simulink library "ros2lib"  (R2022a)
settings: Solver=ode45  StartTime=0.0  StopTime=10.0  RelTol=1e-3  EnableMultiTasking=on
undefined symbols (not defined in the file or in its folder): coder, count, data, data_SL_Info, datatype, encoding, encoding_SL_Info, fields, fields_SL_Info, height, name, name_SL_Info, offset, point_step, ros, row_step, width
settings Model: Creator=The MathWorks, Inc.  LastModifiedBy=The MathWorks, Inc.
settings SolverCC: AlgebraicLoopSolver=TrustRegion  MaxZcPerStep=1
settings DataIOCC: LimitDataPoints=on  SaveFormat=Array  ReturnWorkspaceOutputs=off
settings OptimizationCC: LifeSpan=inf
settings DebuggingCC: SolverPrmCheckMsg=warning  UnconnectedInputMsg=warning  UnconnectedOutputMsg=warning  UnconnectedLineMsg=warning  AllowSymbolicDim=off  PregeneratedLibrarySubsystemCodeDiagnostic=none  SFUnexpectedBacktrackingDiag=warning  SFNoUnconditionalDefaultTransitionDiag=warning  SFExecutionAtInitializationDiag=none  SFMachineParentedDataDiag=warning  ArithmeticOperatorsInVariantConditions=warning
settings HardwareCC: ProdBitPerPointer=32  ProdBitPerSizeT=32  ProdBitPerPtrDiffT=32  ProdLargestAtomicFloat=None  ProdIntDivRoundTo=Undefined  ProdEndianess=Unspecified  ProdWordSize=32  ProdHWDeviceType=32-bit Generic
settings ModelReferenceCC: PropagateSignalLabelsOutOfModel=off
settings SFSimCC: SimUseLocalCustomCode=off
settings RTWCC: RTWUseLocalCustomCode=off  DLArmComputeVersion=19.05
settings CodeAppCC: StateflowObjectComments=on
settings GRTTargetCC: TargetLangStandard=C89/C90 (ANSI)
settings ConfigComp: CovScope=ReferencedModels  CovMetricSettings=dw  CovSaveCumulativeToWorkspaceVar=on  CovSaveSingleToWorkspaceVar=on  CovExternalEMLEnable=off  CovSFcnEnable=off

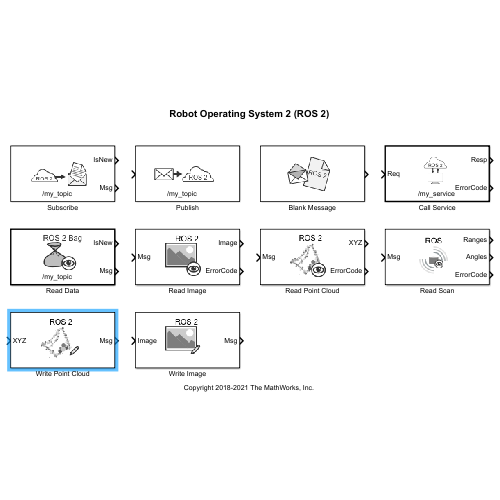
[thumbnail: Simulink's stored preview of the top-level diagram]
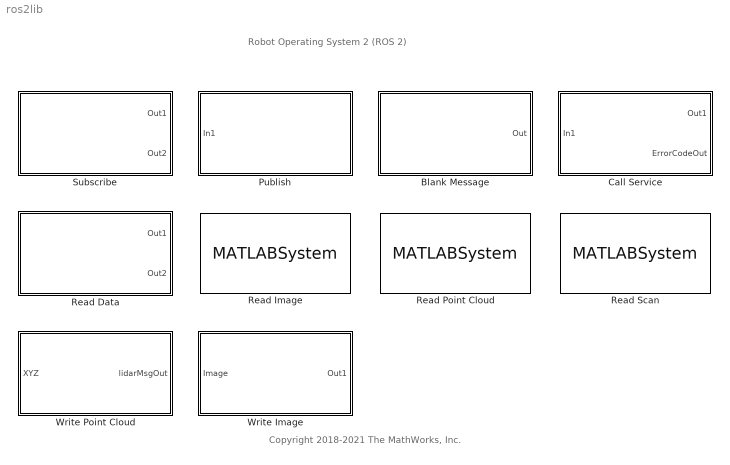
== system ros2lib ==
  note: Copyright 2018-2021 The MathWorks, Inc.
  note: Robot Operating System 2 (ROS 2)
  Blank Message : Subsystem  LoadFcn=ros.slros2.internal.block.MessageBlockMask.messageLoadFcn(gcb);  InitFcn=ros.slros.internal.block.errorIfBlocksConflict(bdroot(gcb));  mask(ROS2 Blank Message){messageClass=Message, entityType=geometry_msgs/Point, messageType=geometry_msgs/Point, SampleTime=inf}
      mask prompts: messageClass "ros:slros:blockmask:MessageClassPrompt"; entityType "ros:slros:blockmask:TypePrompt"; messageType "ros:slros:blockmask:FullTypePrompt"; SampleTime "Simulink:blkprm_prompts:AllSrcBlksSampleTime"
      mask help: ros:slros2:blockmask:BlankMsgDescription
      mask init:
      | ros.slros2.internal.block.MessageBlockMask.dispatch('maskInitialize', gcb);
      settings: ModelCloseFcn=ros.slros2.internal.bus.Util.clearSLBusesInGlobalScope(gcb);
      mask Help: eval('ros.slros.internal.helpview(''ros2BlankMsgBlock'')');
      mask TypeOptions messageClass: ros:slros:blockmask:MessageType_Msg | ros:slros:blockmask:MessageType_SrvReq | ros:slros:blockmask:MessageType_SrvResp
      mask Callback messageClass: ros.slros2.internal.block.MessageBlockMask.dispatch('messageClassChange', gcb);
      mask Callback entityType: ros.slros2.internal.block.MessageBlockMask.dispatch('entityTypeEdit', gcb);
      mask TypeOptions SampleTime: Constant/SampleTime
      mask DialogControl messageClass Prompt: Class:
      mask DialogControl entityType Prompt: Type:
      mask DialogControl id_msgTypeSelectBtn Prompt: ros:slros:blockmask:SelectPrompt
      mask DialogControl id_msgTypeSelectBtn Callback: ros.slros2.internal.block.MessageBlockMask.dispatch('selectButtonPressed', gcb);
      mask DialogControl messageType Prompt: Fully resolved type:
      mask DialogControl SampleTime Prompt: Sample time:
      mask Display: color('black');
  Call Service : Subsystem  LoadFcn=ros.slros2.internal.block.ServiceCallBlockMask.messageLoadFcn(gcb);  InitFcn=ros.slros.internal.block.errorIfBlocksConflict(bdroot(gcb));  TreatAsAtomicUnit=on  mask(ROS2 Call Service){topicSource=Select from ROS network, service=/my_service, serviceType=std_srvs/Empty, connectionTimeout=5, ShowErrorCodeOutput=on, legacyBusStruct=off, QOSHistory=Keep last, QOSDepth=1, QOSReliability=Reliable, QOSDurability=Volatile}
      mask prompts: topicSource "ros:slros:svccaller:SourcePrompt"; service "ros:slros:svccaller:NamePrompt"; serviceType "ros:slros:svccaller:TypePrompt"; connectionTimeout "ros:slros:svccaller:ConnectionTimeoutPrompt"; ShowErrorCodeOutput "ros:slros:blockmask:ShowErrorCodePrompt"; legacyBusStruct "Use legacy bus structure"; QOSHistory "ros:slros2:blockmask:QOSHistoryPrompt"; QOSDepth "ros:slros2:blockmask:QOSDepthPrompt"; QOSReliability "ros:slros2:blockmask:QOSReliabilityPrompt"; QOSDurability "ros:slros2:blockmask:QOSDurabilityPrompt"
      mask help: ros:slros2:blockmask:ServiceCallerDescription
      mask init:
      | ros.slros2.internal.block.ServiceCallBlockMask.dispatch('maskInitialize', gcb);
      settings: ModelCloseFcn=ros.slros2.internal.bus.Util.clearSLBusesInGlobalScope(gcb);
      mask Help: eval('ros.slros.internal.helpview(''ros2CallServiceBlock'')');
      mask TypeOptions topicSource: ros:slros:blockmask:TopicSourceFromNetwork | ros:slros:blockmask:TopicSourceSpecifyOwn
      mask Callback topicSource: ros.slros2.internal.block.ServiceCallBlockMask.dispatch('serviceSourceSelect', gcb);
      mask Callback service: ros.slros2.internal.block.ServiceCallBlockMask.dispatch('serviceEdit', gcb);
      mask Callback connectionTimeout: ros.slros2.internal.block.ServiceCallBlockMask.dispatch('connectionTimeoutEdit', gcb);
      mask TypeOptions QOSHistory: ServiceCaller/QOSHistory
      mask Callback QOSHistory: ros.slros2.internal.block.QOSSettingsMask.qosHistorySelect(gcb);
      mask TypeOptions QOSDepth: ServiceCaller/QOSDepth
      mask TypeOptions QOSReliability: ServiceCaller/QOSReliability
      mask TypeOptions QOSDurability: ServiceCaller/QOSDurability
      mask DialogControl id_netAddrLink Prompt: ros:slros2:blockmask:ConfigNetworkAddrLinkText
      mask DialogControl id_netAddrLink Callback: ros.slros2.internal.block.SubscribeBlockMask.dispatch('configureNetworkAddrDlg', gcb);
      mask DialogControl Container6 Prompt: ros:slros2:blockmask:PubSubMainTab
      mask DialogControl topicSource Prompt: Source:
      mask DialogControl service Prompt: Name:
      mask DialogControl id_topicSelectBtn Prompt: ros:slros:blockmask:SelectPrompt
      mask DialogControl id_topicSelectBtn Callback: ros.slros2.internal.block.ServiceCallBlockMask.dispatch('serviceSelect', gcb, 'ros.slros2.internal.dlg.ServiceSelector');
      mask DialogControl serviceType Prompt: Type:
      mask DialogControl id_msgTypeSelectBtn Prompt: ros:slros:blockmask:SelectPrompt
      mask DialogControl id_msgTypeSelectBtn Callback: ros.slros2.internal.block.ServiceCallBlockMask.dispatch('serviceTypeSelect', gcb, 'ros.slros2.internal.dlg.ServiceTypeSelector');
      mask DialogControl connectionTimeout Prompt: Connection timeout:
      mask DialogControl ShowErrorCodeOutput Prompt: Show ErrorCode output port
      mask DialogControl id_cgContainer Prompt: ros:slros2:blockmask:PubSubQOSTab
      mask DialogControl QOSHistory Prompt: History:
      mask DialogControl QOSDepth Prompt: Depth:
      mask DialogControl QOSReliability Prompt: Reliability:
      mask DialogControl QOSDurability Prompt: Durability:
      mask Display:
      | color('black');
      | text(0.5, 0.15, '/my_service', 'horizontalAlignment', 'center');
      | port_label('input', 1, 'Req');
      | port_label('output', 1, 'Resp');
      | port_label('output', 2, 'ErrorCode');
  Publish : Subsystem  LoadFcn=ros.slros2.internal.block.PublishBlockMask.messageLoadFcn(gcb);  InitFcn=ros.slros.internal.block.errorIfBlocksConflict(bdroot(gcb));  mask(ROS2 Publish){topicSource=Select from ROS network, topic=/my_topic, messageType=geometry_msgs/Point, QOSHistory=Keep last, QOSDepth=1, QOSReliability=Reliable, QOSDurability=Volatile}
      mask prompts: topicSource "ros:slros:blockmask:TopicSourcePrompt"; topic "ros:slros:blockmask:TopicPrompt"; messageType "ros:slros:blockmask:MessageTypePrompt"; QOSHistory "ros:slros2:blockmask:QOSHistoryPrompt"; QOSDepth "ros:slros2:blockmask:QOSDepthPrompt"; QOSReliability "ros:slros2:blockmask:QOSReliabilityPrompt"; QOSDurability "ros:slros2:blockmask:QOSDurabilityPrompt"
      mask help: ros:slros:blockmask:PublisherDescription
      mask init:
      | ros.slros2.internal.block.PublishBlockMask.dispatch('maskInitialize', gcb);
      settings: ModelCloseFcn=ros.slros2.internal.bus.Util.clearSLBusesInGlobalScope(gcb);
      mask Help: eval('ros.slros.internal.helpview(''ros2PublishBlock'')');
      mask TypeOptions topicSource: ros:slros2:blockmask:TopicSourceFromNetwork | ros:slros2:blockmask:TopicSourceSpecifyOwn
      mask Callback topicSource: ros.slros2.internal.block.PublishBlockMask.dispatch('topicSourceSelect', gcb);
      mask Callback topic: ros.slros2.internal.block.PublishBlockMask.dispatch('topicEdit', gcb);
      mask Callback messageType: ros.slros2.internal.block.PublishBlockMask.dispatch('messageTypeEdit', gcb);
      mask TypeOptions QOSHistory: SinkBlock/QOSHistory
      mask Callback QOSHistory: ros.slros2.internal.block.QOSSettingsMask.qosHistorySelect(gcb);
      mask TypeOptions QOSDepth: SinkBlock/QOSDepth
      mask TypeOptions QOSReliability: SinkBlock/QOSReliability
      mask TypeOptions QOSDurability: SinkBlock/QOSDurability
      mask DialogControl id_netAddrLink Prompt: ros:slros2:blockmask:ConfigNetworkAddrLinkText
      mask DialogControl id_netAddrLink Callback: ros.slros2.internal.block.PublishBlockMask.dispatch('configureNetworkAddrDlg', gcb);
      mask DialogControl Container13 Prompt: ros:slros2:blockmask:PubSubMainTab
      mask DialogControl topicSource Prompt: Topic source:
      mask DialogControl topic Prompt: Topic:
      mask DialogControl id_topicSelectBtn Prompt: ros:slros:blockmask:SelectPrompt
      mask DialogControl id_topicSelectBtn Callback: ros.slros2.internal.block.PublishBlockMask.dispatch('topicSelect', gcb, 'ros.slros2.internal.dlg.TopicSelector');
      mask DialogControl messageType Prompt: Message type:
      mask DialogControl id_msgTypeSelectBtn Prompt: ros:slros:blockmask:SelectPrompt
      mask DialogControl id_msgTypeSelectBtn Callback: ros.slros2.internal.block.PublishBlockMask.dispatch('messageTypeSelect', gcb, 'ros.slros2.internal.dlg.MessageTypeSelector');
      mask DialogControl id_cgContainer Prompt: ros:slros2:blockmask:PubSubQOSTab
      mask DialogControl QOSHistory Prompt: History:
      mask DialogControl QOSDepth Prompt: Depth:
      mask DialogControl QOSReliability Prompt: Reliability:
      mask DialogControl QOSDurability Prompt: Durability:
      mask Display:
      | color('black');
      | text(0.45, 0.15, '/my_topic', 'horizontalAlignment', 'center');
  Read Data : Subsystem  InitFcn=ros.slros.internal.block.errorIfBlocksConflict(bdroot(gcb));  TreatAsAtomicUnit=on  mask(Read Data from ROS2 Bag){topic=/my_topic, sampleTime=-1, logfileType=rosbag2, modelName=ros2lib, msgType=}
      mask prompts: topic "ros:slros:readlog:TopicPrompt"; sampleTime "ros:slros:blockmask:SampleTimePrompt"
      mask help: ros:slros:readlog:ReadDataDescription
      mask init:
      | ros.slros.internal.block.ReadDataBlockMask.blockInitFcn(gcb);
      settings: ModelCloseFcn=ros.slros.internal.block.ReadDataBlockMask.modelCloseFcn(gcb);
      mask Help: eval('ros.slros.internal.helpview(''ros2ReadDataBlock'')');
      mask TypeOptions topic: SourceBlock/Topic
      mask TypeOptions sampleTime: SourceBlock/SampleTime
      mask TypeOptions logfileType: SourceBlock/LogfileType
      mask TypeOptions modelName: SourceBlock/ModelName
      mask TypeOptions msgType: SourceBlock/MsgType
      mask DialogControl id_logDataLink Prompt: ros:slros:readlog:LoadDataPrompt
      mask DialogControl id_logDataLink Callback: ros.slros.internal.block.ReadDataBlockMask.loadLogfileLink(gcb)
      mask DialogControl topic Prompt: Topic:
      mask DialogControl id_topicSelectBtn Prompt: ros:slros:readlog:SelectPrompt
      mask DialogControl id_topicSelectBtn Callback: ros.slros.internal.block.ReadDataBlockMask.topicSelectButton(gcb)
      mask DialogControl sampleTime Prompt: Sample time:
      mask Display:
      | color('black');
      | text(0.45, 0.15, '/my_topic', 'horizontalAlignment', 'center');
      | port_label('output', 1, 'IsNew');
      | port_label('output', 2, 'Msg');
  Read Image : MATLABSystem  InitFcn=ros.slros.internal.block.errorIfBlocksConflict(bdroot(gcb));  System=ros.slros2.internal.block.ReadImage  MaximumImageSize=[ 2000, 2000 ]  ImageEncoding=rgb8  ShowAlphaOutput=off  ShowErrorCodeOutput=on  VariableSizeOutputs=off
      mask Type: ros.slros2.internal.block.ReadImage
      mask Display:
      | port_label('input',1,'Msg');
      | port_label('output',1,'Image');
      | port_label('output',2,'ErrorCode');
  Read Point Cloud : MATLABSystem  InitFcn=ros.slros.internal.block.errorIfBlocksConflict(bdroot(gcb));  System=ros.slros2.internal.block.ReadPointCloud  MaximumPointCloudSize=[480, 640]  PreserveStructure=off  ShowRGBOutput=off  ShowIntensityOutput=off  ShowErrorCodeOutput=on  VariableSizeOutputs=off
      mask Type: ros.slros2.internal.block.ReadPointCloud
      mask Display:
      | port_label('input',1,'Msg');
      | port_label('output',1,'XYZ');
      | port_label('output',2,'ErrorCode');
  Read Scan : MATLABSystem  InitFcn=ros.slros.internal.block.errorIfBlocksConflict(bdroot(gcb));  System=ros.slros2.internal.block.ReadScan  MaximumArrayLength=100  ShowAnglesOutput=on  ShowIntensityOutput=off  ShowErrorCodeOutput=on  VariableSizeOutputs=off
      mask Type: ros.slros2.internal.block.ReadScan
      mask Display:
      | port_label('input',1,'Msg');
      | port_label('output',1,'Ranges');
      | port_label('output',2,'Angles');
      | port_label('output',3,'ErrorCode');
  Subscribe : Subsystem  LoadFcn=ros.slros2.internal.block.SubscribeBlockMask.messageLoadFcn(gcb);  InitFcn=ros.slros.internal.block.errorIfBlocksConflict(bdroot(gcb));  mask(ROS2 Subscribe){topicSource=Select from ROS network, topic=/my_topic, messageType=geometry_msgs/Point, sampleTime=-1, QOSHistory=Keep last, QOSDepth=1, QOSReliability=Reliable, QOSDurability=Volatile}
      mask prompts: topicSource "ros:slros:blockmask:TopicSourcePrompt"; topic "ros:slros:blockmask:TopicPrompt"; messageType "ros:slros:blockmask:MessageTypePrompt"; sampleTime "ros:slros:blockmask:SampleTimePrompt"; QOSHistory "ros:slros2:blockmask:QOSHistoryPrompt"; QOSDepth "ros:slros2:blockmask:QOSDepthPrompt"; QOSReliability "ros:slros2:blockmask:QOSReliabilityPrompt"; QOSDurability "ros:slros2:blockmask:QOSDurabilityPrompt"
      mask help: ros:slros:blockmask:SubscriberDescription
      mask init:
      | ros.slros2.internal.block.SubscribeBlockMask.dispatch('maskInitialize', gcb);
      settings: ModelCloseFcn=ros.slros2.internal.bus.Util.clearSLBusesInGlobalScope(gcb);
      mask Help: eval('ros.slros.internal.helpview(''ros2SubscribeBlock'')');
      mask TypeOptions topicSource: ros:slros2:blockmask:TopicSourceFromNetwork | ros:slros2:blockmask:TopicSourceSpecifyOwn
      mask Callback topicSource: ros.slros2.internal.block.SubscribeBlockMask.dispatch('topicSourceSelect', gcb);
      mask Callback topic: ros.slros2.internal.block.SubscribeBlockMask.dispatch('topicEdit', gcb);
      mask Callback messageType: ros.slros2.internal.block.SubscribeBlockMask.dispatch('messageTypeEdit', gcb);
      mask TypeOptions sampleTime: Constant/SampleTime
      mask TypeOptions QOSHistory: SourceBlock/QOSHistory
      mask Callback QOSHistory: ros.slros2.internal.block.QOSSettingsMask.qosHistorySelect(gcb);
      mask TypeOptions QOSDepth: SourceBlock/QOSDepth
      mask TypeOptions QOSReliability: SourceBlock/QOSReliability
      mask TypeOptions QOSDurability: SourceBlock/QOSDurability
      mask DialogControl id_netAddrLink Prompt: ros:slros2:blockmask:ConfigNetworkAddrLinkText
      mask DialogControl id_netAddrLink Callback: ros.slros2.internal.block.SubscribeBlockMask.dispatch('configureNetworkAddrDlg', gcb);
      mask DialogControl Container13 Prompt: ros:slros2:blockmask:PubSubMainTab
      mask DialogControl topicSource Prompt: Topic source:
      mask DialogControl topic Prompt: Topic:
      mask DialogControl id_topicSelectBtn Prompt: ros:slros:blockmask:SelectPrompt
      mask DialogControl id_topicSelectBtn Callback: ros.slros2.internal.block.SubscribeBlockMask.dispatch('topicSelect', gcb, 'ros.slros2.internal.dlg.TopicSelector');
      mask DialogControl messageType Prompt: Message type:
      mask DialogControl id_msgTypeSelectBtn Prompt: ros:slros:blockmask:SelectPrompt
      mask DialogControl id_msgTypeSelectBtn Callback: ros.slros2.internal.block.SubscribeBlockMask.dispatch('messageTypeSelect', gcb, 'ros.slros2.internal.dlg.MessageTypeSelector');
      mask DialogControl sampleTime Prompt: Sample time:
      mask DialogControl id_cgContainer Prompt: ros:slros2:blockmask:PubSubQOSTab
      mask DialogControl QOSHistory Prompt: History:
      mask DialogControl QOSDepth Prompt: Depth:
      mask DialogControl QOSReliability Prompt: Reliability:
      mask DialogControl QOSDurability Prompt: Durability:
      mask Display:
      | color('black');
      | text(0.45, 0.15, '/my_topic', 'horizontalAlignment', 'center');
      | port_label('output', 1, 'IsNew');
      | port_label('output', 2, 'Msg');
  Write Image : Subsystem  InitFcn=|  mask(ROS2 Write Image){ImageEncoding=rgb8, EncodingStruct=ros.msg.sensor_msgs.internal.ImageEncoding.info(coder.const('rgb8')), HasAlpha=off, messageType=sensor_msgs/Image}
      | ros.slros.internal.block.errorIfBlocksConflict(bdroot(gcb));
      | ros.slros2.internal.block.WriteImageBlockMask.dispatch('maskInitialize', gcb);
      mask prompts: ImageEncoding "ros:slros2:blockmask:ImageEncodingPrompt"
      mask init:
      | ros.slros2.internal.block.WriteImageBlockMask.dispatch('maskInitialize', gcb);
      mask Help: eval('ros.slros.internal.helpview(''ros2WriteImBlock'')');
      mask TypeOptions ImageEncoding: rgb8 | rgba8 | rgb16 | rgba16 | bgr8 | bgra8 | bgr16 | bgra16 | mono8 | mono16 | 32fc1 | 32fc2 | 32fc3 | 32fc4 | 64fc1 | 64fc2 | 64fc3 | 64fc4 | 8uc1 | 8uc2 | 8uc3 | 8uc4 | 8sc1 | 8sc2 | 8sc3 | 8sc4 | 16uc1 | 16uc2 | 16uc3 | 16uc4 | 16sc1 | 16sc2 | 16sc3 | 16sc4 | 32sc1 | 32sc2 | 32sc3 | 32sc4
      mask DialogControl DescGroupVar Prompt: ros:slros2:blockmask:WriteImageTitle
      mask DialogControl DescTextVar Prompt: ros:slros2:blockmask:WriteImageDescription
      mask DialogControl Settings Prompt: ros:slros2:blockmask:ImagePropertiesPrompt
      mask DialogControl ImageEncoding Prompt: Image encoding:
      mask Display: port_label('input',1,'Image');port_label('output',1,'Msg');
  Write Point Cloud : Subsystem  InitFcn=|  mask(ROS2 Write Point Cloud){Encoding=none, HasRGB=false, HasAlpha=false, FieldNamesStruct=struct('x', 'single', 'y', 'single', 'z', 'single'), messageType=sensor_msgs/PointCloud2}
      | ros.slros.internal.block.errorIfBlocksConflict(bdroot(gcb));
      | ros.slros2.internal.block.WritePointCloudBlockMask.dispatch('maskInitialize', gcb);
      mask prompts: Encoding "ros:slros2:blockmask:SelectRGBInputPrompt"
      mask init:
      | ros.slros2.internal.block.WritePointCloudBlockMask.dispatch('maskInitialize', gcb);
      mask Help: eval('ros.slros.internal.helpview(''ros2WritePCBlock'')');
      mask TypeOptions Encoding: none | rgb | rgba
      mask DialogControl DescGroupVar Prompt: ros:slros2:blockmask:WritePointCloudTitle
      mask DialogControl DescTextVar Prompt: ros:slros2:blockmask:WritePointCloudDescription
      mask DialogControl ParameterGroupVar Prompt: ros:slros2:blockmask:InputConfiguration
      mask DialogControl Encoding Prompt: Select color field
      mask Display: port_label('input',1,'XYZ');port_label('output',1,'Msg');

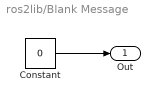
== system ros2lib/Blank Message ==
  Constant : Constant  Value=0  OutDataTypeStr=Bus: SL_Bus_geometry_msgs_Point  SampleTime=SampleTime  LockScale=on
  Out : Outport  VectorParamsAs1DForOutWhenUnconnected=off  LockScale=on
  wires:
  Constant/1 -> Out/1

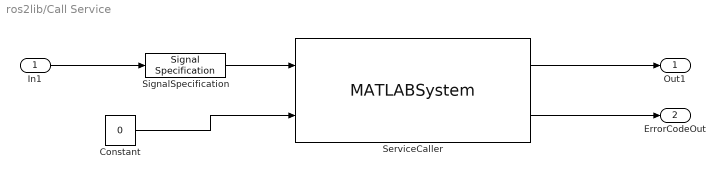
== system ros2lib/Call Service ==
  In1 : Inport
  Constant : Constant  Value=0  VectorParams1D=off  OutDataTypeStr=Bus: SL_Bus_std_srvs_EmptyResponse  SampleTime=-1
  ServiceCaller : MATLABSystem  System=ros.slros2.internal.block.ServiceCaller  QOSHistory=Keep last  QOSDepth=QOSDepth  QOSReliability=Reliable  QOSDurability=Volatile  ServiceName=/my_service  ServiceType=std_srvs/Empty  ConnectionTimeout=5  IsPersistentConnection=off  SLInputBusName=SL_Bus_std_srvs_EmptyRequest  SLOutputBusName=SL_Bus_std_srvs_EmptyResponse  ModelName=ros2lib  BlockId=ServCall_ros2lib_179
      mask Type: ros.slros2.internal.block.ServiceCaller
      mask Display:
      | disp('ServiceCaller');
      | port_label('input',1,'inputbusstruct');
      | port_label('input',2,'outputbusstruct');
      | port_label('output',1,'respMsg');
      | port_label('output',2,'errorCode');
  SignalSpecification : SignalSpecification  OutDataTypeStr=Bus: SL_Bus_std_srvs_EmptyRequest  BusOutputAsStruct=on
      settings: LockScale=on
  Out1 : Outport
  ErrorCodeOut : Outport  Port=2
  wires:
  ServiceCaller/2 -> ErrorCodeOut/1
  Constant/1 -> ServiceCaller/2
  ServiceCaller/1 -> Out1/1
  In1/1 -> SignalSpecification/1
  SignalSpecification/1 -> ServiceCaller/1

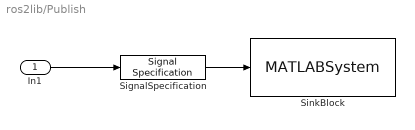
== system ros2lib/Publish ==
  In1 : Inport  LockScale=on
  SignalSpecification : SignalSpecification  OutDataTypeStr=Bus: SL_Bus_geometry_msgs_Point  BusOutputAsStruct=on
      settings: LockScale=on
  SinkBlock : MATLABSystem  System=ros.slros2.internal.block.Publisher  QOSHistory=Keep last  QOSDepth=QOSDepth  QOSReliability=Reliable  QOSDurability=Volatile  ROSTopic=/my_topic  ROSMessageType=geometry_msgs/Point  SLBusName=SL_Bus_geometry_msgs_Point  ModelName=ros2lib  BlockId=Pub_ros2lib_156
      mask Type: ros.slros2.internal.block.Publisher
      mask Display:
      | disp('Publisher');
      | port_label('input',1,'busstruct');
  wires:
  SignalSpecification/1 -> SinkBlock/1
  In1/1 -> SignalSpecification/1

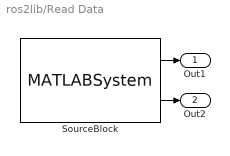
== system ros2lib/Read Data ==
  SourceBlock : MATLABSystem  System=ros.slros2.internal.block.ReadData  LogfileType=rosbag2  Topic=/my_topic  SampleTime=-1  ModelName=ros2lib
      mask Type: ros.slros2.internal.block.ReadData
      mask Display:
      | disp('ReadData');
      | port_label('output',1,'isNew');
      | port_label('output',2,'msg');
  Out1 : Outport
  Out2 : Outport  Port=2
  wires:
  SourceBlock/2 -> Out2/1
  SourceBlock/1 -> Out1/1

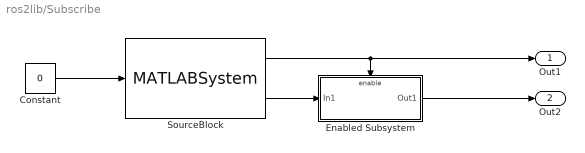
== system ros2lib/Subscribe ==
  Constant : Constant  Value=0  OutDataTypeStr=Bus: SL_Bus_geometry_msgs_Point  SampleTime=sampleTime  LockScale=on
  Enabled Subsystem : Subsystem  TreatAsAtomicUnit=on
  SourceBlock : MATLABSystem  System=ros.slros2.internal.block.Subscriber  QOSHistory=Keep last  QOSDepth=QOSDepth  QOSReliability=Reliable  QOSDurability=Volatile  ROSTopic=/my_topic  ROSMessageType=geometry_msgs/Point  SLBusName=SL_Bus_geometry_msgs_Point  ModelName=ros2lib  BlockId=Sub_ros2lib_139
      mask Type: ros.slros2.internal.block.Subscriber
      mask Display:
      | disp('Subscriber');
      | port_label('input',1,'busstruct');
      | port_label('output',1,'isNewData');
      | port_label('output',2,'msg');
  Out1 : Outport  VectorParamsAs1DForOutWhenUnconnected=off
  Out2 : Outport  Port=2  VectorParamsAs1DForOutWhenUnconnected=off
  wires:
  SourceBlock/1 -> Enabled Subsystem/Enable, Out1/1
  SourceBlock/2 -> Enabled Subsystem/1(In1)
  Constant/1 -> SourceBlock/1
  Enabled Subsystem/1(Out1) -> Out2/1

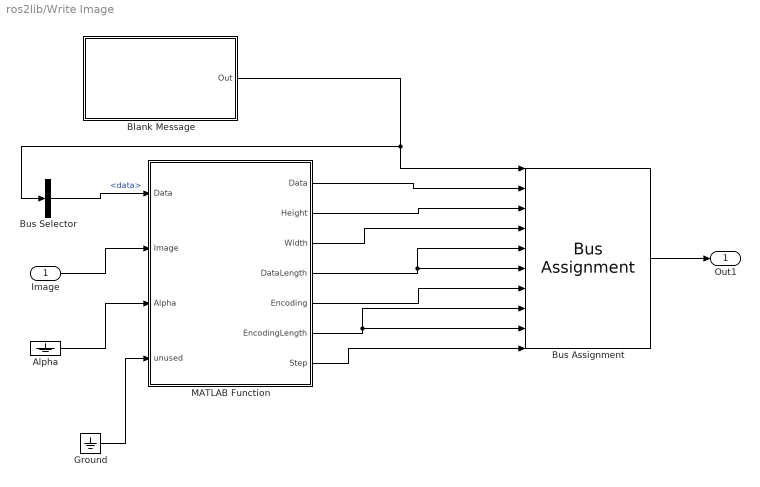
== system ros2lib/Write Image ==
  Image : Inport
  Alpha : Ground
  Blank Message : Subsystem  LoadFcn=ros.slros2.internal.block.MessageBlockMask.messageLoadFcn(gcb);  InitFcn=ros.slros.internal.block.errorIfBlocksConflict(bdroot(gcb));  mask(ROS2 Blank Message){messageClass=Message, entityType=sensor_msgs/Image, messageType=sensor_msgs/Image, SampleTime=inf}
      mask prompts: messageClass "ros:slros:blockmask:MessageClassPrompt"; entityType "ros:slros:blockmask:TypePrompt"; messageType "ros:slros:blockmask:FullTypePrompt"; SampleTime "Simulink:blkprm_prompts:AllSrcBlksSampleTime"
      mask help: ros:slros2:blockmask:BlankMsgDescription
      mask init:
      | ros.slros2.internal.block.MessageBlockMask.dispatch('maskInitialize', gcb);
      settings: ModelCloseFcn=ros.slros2.internal.bus.Util.clearSLBusesInGlobalScope();
      mask Help: eval('ros.slros.internal.helpview(''ros2BlankMsgBlock'')');
      mask TypeOptions messageClass: ros:slros:blockmask:MessageType_Msg | ros:slros:blockmask:MessageType_SrvReq | ros:slros:blockmask:MessageType_SrvResp
      mask Callback messageClass: ros.slros2.internal.block.MessageBlockMask.dispatch('messageClassChange', gcb);
      mask Callback entityType: ros.slros2.internal.block.MessageBlockMask.dispatch('entityTypeEdit', gcb);
      mask TypeOptions SampleTime: Constant/SampleTime
      mask DialogControl messageClass Prompt: Class:
      mask DialogControl entityType Prompt: Type:
      mask DialogControl id_msgTypeSelectBtn Prompt: ros:slros:blockmask:SelectPrompt
      mask DialogControl id_msgTypeSelectBtn Callback: ros.slros2.internal.block.MessageBlockMask.dispatch('selectButtonPressed', gcb);
      mask DialogControl messageType Prompt: Fully resolved type:
      mask DialogControl SampleTime Prompt: Sample time:
      mask Display: color('black');
  Bus Assignment : BusAssignment  AssignedSignals=data,height,width,data_SL_Info.CurrentLength,data_SL_Info.ReceivedLength,encoding,encoding_SL_Info.CurrentLength,encoding_SL_Info.ReceivedLength,step
  Bus Selector : BusSelector  OutputSignals=data
  Ground : Ground
  MATLAB Function : MATLAB Function  TreatAsAtomicUnit=on
  Out1 : Outport
  wires:
  MATLAB Function/1(Data) -> Bus Assignment/2
  MATLAB Function/3(Width) -> Bus Assignment/4
  MATLAB Function/5(Encoding) -> Bus Assignment/7
  Blank Message/1(Out) -> Bus Selector/1, Bus Assignment/1
  Bus Assignment/1 -> Out1/1
  MATLAB Function/2(Height) -> Bus Assignment/3
  Bus Selector/1 -> MATLAB Function/1("Data ")  "<data>"
  MATLAB Function/7(Step) -> Bus Assignment/10
  MATLAB Function/6(EncodingLength) -> Bus Assignment/8, Bus Assignment/9
  MATLAB Function/4(DataLength) -> Bus Assignment/5, Bus Assignment/6
  Image/1 -> MATLAB Function/2(Image)
  Alpha/1 -> MATLAB Function/3(Alpha)
  Ground/1 -> MATLAB Function/4(unused)

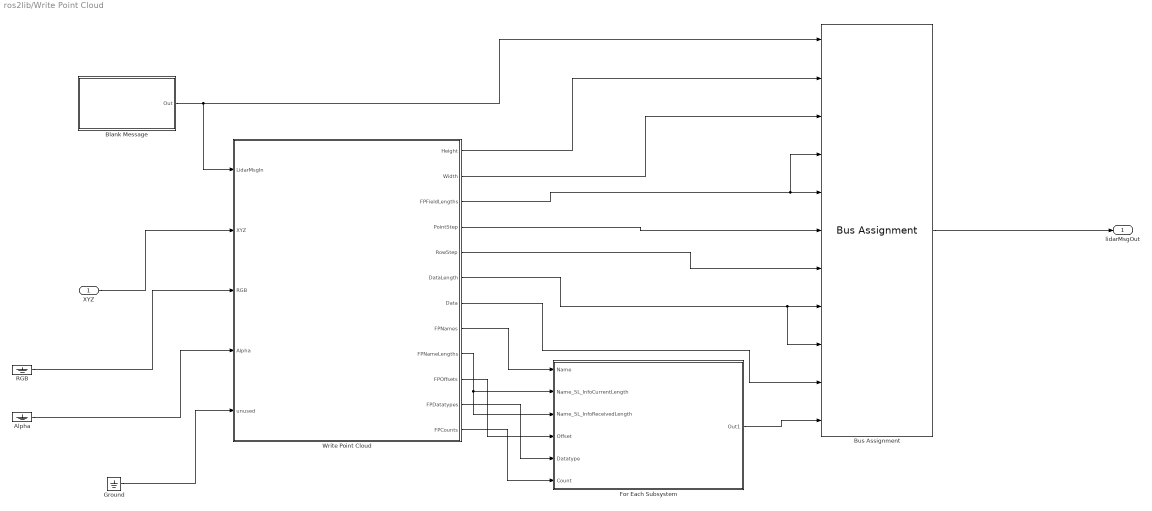
== system ros2lib/Write Point Cloud ==
  XYZ : Inport
  Alpha : Ground
  Blank Message : Subsystem  LoadFcn=ros.slros2.internal.block.MessageBlockMask.messageLoadFcn(gcb);  InitFcn=ros.slros.internal.block.errorIfBlocksConflict(bdroot(gcb));  mask(ROS2 Blank Message){messageClass=Message, entityType=sensor_msgs/PointCloud2, messageType=sensor_msgs/PointCloud2, SampleTime=inf}
      mask prompts: messageClass "ros:slros:blockmask:MessageClassPrompt"; entityType "ros:slros:blockmask:TypePrompt"; messageType "ros:slros:blockmask:FullTypePrompt"; SampleTime "Simulink:blkprm_prompts:AllSrcBlksSampleTime"
      mask help: ros:slros2:blockmask:BlankMsgDescription
      mask init:
      | ros.slros2.internal.block.MessageBlockMask.dispatch('maskInitialize', gcb);
      settings: ModelCloseFcn=ros.slros2.internal.bus.Util.clearSLBusesInGlobalScope();
      mask Help: eval('ros.slros.internal.helpview(''ros2BlankMsgBlock'')');
      mask TypeOptions messageClass: ros:slros:blockmask:MessageType_Msg | ros:slros:blockmask:MessageType_SrvReq | ros:slros:blockmask:MessageType_SrvResp
      mask Callback messageClass: ros.slros2.internal.block.MessageBlockMask.dispatch('messageClassChange', gcb);
      mask Callback entityType: ros.slros2.internal.block.MessageBlockMask.dispatch('entityTypeEdit', gcb);
      mask TypeOptions SampleTime: Constant/SampleTime
      mask DialogControl messageClass Prompt: Class:
      mask DialogControl entityType Prompt: Type:
      mask DialogControl id_msgTypeSelectBtn Prompt: ros:slros:blockmask:SelectPrompt
      mask DialogControl id_msgTypeSelectBtn Callback: ros.slros2.internal.block.MessageBlockMask.dispatch('selectButtonPressed', gcb);
      mask DialogControl messageType Prompt: Fully resolved type:
      mask DialogControl SampleTime Prompt: Sample time:
      mask Display: color('black');
  Bus Assignment : BusAssignment  AssignedSignals=height,width,fields_SL_Info.CurrentLength,fields_SL_Info.ReceivedLength,point_step,row_step,data_SL_Info.CurrentLength,data_SL_Info.ReceivedLength,data,fields
  For Each Subsystem : Subsystem  TreatAsAtomicUnit=on
  Ground : Ground
  RGB : Ground
  Write Point Cloud : MATLAB Function  TreatAsAtomicUnit=on
  lidarMsgOut : Outport
  wires:
  RGB/1 -> Write Point Cloud/3(RGB)
  XYZ/1 -> Write Point Cloud/2(XYZ)
  Write Point Cloud/3(FPFieldLengths) -> Bus Assignment/4, Bus Assignment/5
  Write Point Cloud/6(DataLength) -> Bus Assignment/9, Bus Assignment/8
  Write Point Cloud/9(FPNameLengths) -> For Each Subsystem/3(Name_SL_InfoReceivedLength), For Each Subsystem/2(Name_SL_InfoCurrentLength)
  Write Point Cloud/8(FPNames) -> For Each Subsystem/1(Name)
  Write Point Cloud/2(Width) -> Bus Assignment/3
  Write Point Cloud/7(Data) -> Bus Assignment/10
  Write Point Cloud/5(RowStep) -> Bus Assignment/7
  Alpha/1 -> Write Point Cloud/4(Alpha)
  For Each Subsystem/1(Out1) -> Bus Assignment/11
  Bus Assignment/1 -> lidarMsgOut/1
  Ground/1 -> Write Point Cloud/5(unused)
  Write Point Cloud/1(Height) -> Bus Assignment/2
  Write Point Cloud/10(FPOffsets) -> For Each Subsystem/4(Offset)
  Write Point Cloud/11(FPDatatypes) -> For Each Subsystem/5(Datatype)
  Blank Message/1(Out) -> Write Point Cloud/1(LidarMsgIn), Bus Assignment/1
  Write Point Cloud/12(FPCounts) -> For Each Subsystem/6(Count)
  Write Point Cloud/4(PointStep) -> Bus Assignment/6

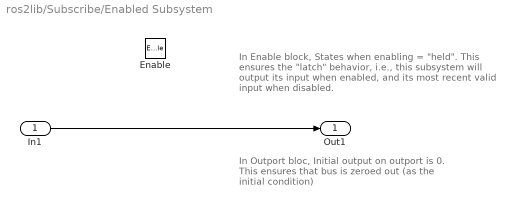
== system ros2lib/Subscribe/Enabled Subsystem ==
  note: In Enable block, States when enabling = "held".
      | This ensures the "latch" behavior, i.e., this subsystem
      | will output its input when enabled, and its most recent
      | valid input when disabled.
  note: In Outport bloc, Initial output on outport is 0.
      | This ensures that bus is zeroed out
      | (as the initial condition)
  In1 : Inport
  Enable : EnablePort
  Out1 : Outport  InitialOutput=0  VectorParamsAs1DForOutWhenUnconnected=off
  wires:
  In1/1 -> Out1/1

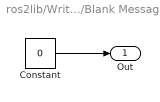
== system ros2lib/Write Image/Blank Message ==
  Constant : Constant  Value=0  OutDataTypeStr=Bus: SL_Bus_sensor_msgs_Image  SampleTime=SampleTime  LockScale=on
  Out : Outport  VectorParamsAs1DForOutWhenUnconnected=off  LockScale=on
  wires:
  Constant/1 -> Out/1

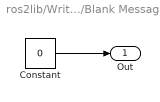
== system ros2lib/Write Point Cloud/Blank Message ==
  Constant : Constant  Value=0  OutDataTypeStr=Bus: SL_Bus_sensor_msgs_PointCloud2  SampleTime=SampleTime  LockScale=on
  Out : Outport  VectorParamsAs1DForOutWhenUnconnected=off  LockScale=on
  wires:
  Constant/1 -> Out/1

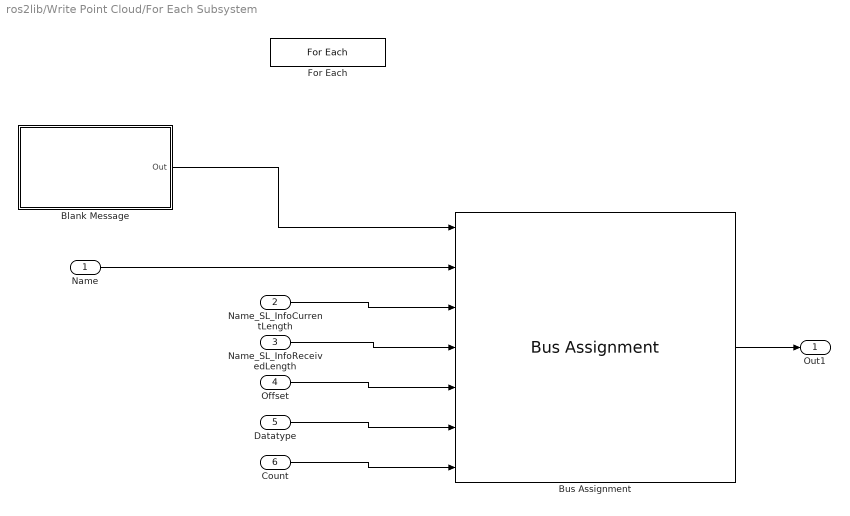
== system ros2lib/Write Point Cloud/For Each Subsystem ==
  Name : Inport  Partition=on  PartitionDimension=1  PartitionWidth=ros.slros.internal.bus.Util.getCurrentFieldLength('sensor_msgs/PointField','name','ros2')  PartitionOffset=0
  Name_SL_InfoCurrentLength : Inport  Port=2  Partition=on  PartitionDimension=1  PartitionWidth=1  PartitionOffset=0
  Name_SL_InfoReceivedLength : Inport  Port=3  Partition=on  PartitionDimension=1  PartitionWidth=1  PartitionOffset=0
  Offset : Inport  Port=4  Partition=on  PartitionDimension=1  PartitionWidth=1  PartitionOffset=0
  Datatype : Inport  Port=5  Partition=on  PartitionDimension=1  PartitionWidth=1  PartitionOffset=0
  Count : Inport  Port=6  Partition=on  PartitionDimension=1  PartitionWidth=1  PartitionOffset=0
  Blank Message : Subsystem  LoadFcn=ros.slros2.internal.block.MessageBlockMask.messageLoadFcn(gcb);  InitFcn=ros.slros.internal.block.errorIfBlocksConflict(bdroot(gcb));  mask(ROS2 Blank Message){messageClass=Message, entityType=sensor_msgs/PointField, messageType=sensor_msgs/PointField, SampleTime=inf}
      mask prompts: messageClass "ros:slros:blockmask:MessageClassPrompt"; entityType "ros:slros:blockmask:TypePrompt"; messageType "ros:slros:blockmask:FullTypePrompt"; SampleTime "Simulink:blkprm_prompts:AllSrcBlksSampleTime"
      mask help: ros:slros2:blockmask:BlankMsgDescription
      mask init:
      | ros.slros2.internal.block.MessageBlockMask.dispatch('maskInitialize', gcb);
      settings: ModelCloseFcn=ros.slros2.internal.bus.Util.clearSLBusesInGlobalScope();
      mask Help: eval('ros.slros.internal.helpview(''ros2BlankMsgBlock'')');
      mask TypeOptions messageClass: ros:slros:blockmask:MessageType_Msg | ros:slros:blockmask:MessageType_SrvReq | ros:slros:blockmask:MessageType_SrvResp
      mask Callback messageClass: ros.slros2.internal.block.MessageBlockMask.dispatch('messageClassChange', gcb);
      mask Callback entityType: ros.slros2.internal.block.MessageBlockMask.dispatch('entityTypeEdit', gcb);
      mask TypeOptions SampleTime: Constant/SampleTime
      mask DialogControl messageClass Prompt: Class:
      mask DialogControl entityType Prompt: Type:
      mask DialogControl id_msgTypeSelectBtn Prompt: ros:slros:blockmask:SelectPrompt
      mask DialogControl id_msgTypeSelectBtn Callback: ros.slros2.internal.block.MessageBlockMask.dispatch('selectButtonPressed', gcb);
      mask DialogControl messageType Prompt: Fully resolved type:
      mask DialogControl SampleTime Prompt: Sample time:
      mask Display: color('black');
  Bus Assignment : BusAssignment  AssignedSignals=name,name_SL_Info.CurrentLength,name_SL_Info.ReceivedLength,offset,datatype,count
  For Each : ForEach  DisableCoverage=on
  Out1 : Outport  ConcatenationDimension=1
  wires:
  Blank Message/1(Out) -> Bus Assignment/1
  Bus Assignment/1 -> Out1/1
  Name_SL_InfoCurrentLength/1 -> Bus Assignment/3
  Name_SL_InfoReceivedLength/1 -> Bus Assignment/4
  Offset/1 -> Bus Assignment/5
  Datatype/1 -> Bus Assignment/6
  Count/1 -> Bus Assignment/7
  Name/1 -> Bus Assignment/2

== system ros2lib/Write Point Cloud/For Each Subsystem/Blank Message ==
  Constant : Constant  Value=0  OutDataTypeStr=Bus: SL_Bus_sensor_msgs_PointField  SampleTime=SampleTime  LockScale=on
  Out : Outport  VectorParamsAs1DForOutWhenUnconnected=off  LockScale=on
  wires:
  Constant/1 -> Out/1

== matlab function ros2lib/Write Image/MATLAB Function ==
  data: Data input; Image input; Alpha input; unused input; Data output; Height output; Width output; DataLength output; Encoding output; EncodingLength output; Step output; EncodingStruct parameter; ImageEncoding parameter; HasAlpha parameter
function [Data, Height, Width, DataLength, Encoding, EncodingLength, Step]...
    = WriteImageFncBlock(Data, Image, Alpha, ~, EncodingStruct, ImageEncoding, HasAlpha)
SelectedEncodingInd = ImageEncoding;
% Image encoding is set to evaluate in the mask,
% so the value is an index.
SelectedEncoding = ros.msg.sensor_msgs.internal.ImageEncoding.AllEncodings{SelectedEncodingInd};
type = EncodingStruct.DataType;
alphaSize = int32(size(Alpha));
imageSize = int32(size(Image));
% check types
if HasAlpha && ~isa(Alpha, type)
coder.internal.error('ros:slros2:image:InvalidAlphaType', SelectedEncoding, type)
elseif HasAlpha && ~ismatrix(Alpha)
coder.internal.error('ros:slros2:image:InvalidAlphaSize')
elseif ~isa(Image, type)
coder.internal.error('ros:slros2:image:InvalidImageType', SelectedEncoding, type)
end
if HasAlpha
    % check sizes
    if ~(imageSize(1) == alphaSize(1) && imageSize(2) == alphaSize(2))
        coder.internal.error('ros:slros2:image:IncompatibleImageAlphaSizes', ...
        fprintf("[%i, %i, %i]", imageSize(1), imageSize(2), imageSize(3)), ...
        fprintf("[%i, %i]", alphaSize(1), alphaSize(2)) )
    end

    ImageInput = cat(3, Image, Alpha);
else
    ImageInput = Image;
end
[Data, Height, Width, DataLength, Encoding, EncodingLength, Step]...
    = ros.internal.block.WriteImageFncBlock(ImageInput, Data, EncodingStruct, SelectedEncodingInd);

== matlab function ros2lib/Write Point Cloud/Write Point Cloud ==
  data: LidarMsgIn input; XYZ input; RGB input; Alpha input; unused input; FieldNamesStruct parameter; HasRGB parameter; HasAlpha parameter; Height output; Width output; FPFieldLengths output; PointStep output; RowStep output; DataLength output; Data output; FPNames output; FPNameLengths output; FPOffsets output; FPDatatypes output; FPCounts output
function [Height, Width, FPFieldLengths, PointStep, ...
    RowStep, DataLength, Data, FPNames,...
    FPNameLengths, FPOffsets, FPDatatypes, FPCounts] ...
    = WritePointCloudFncBlock(LidarMsgIn, XYZ, RGB, Alpha, ~, FieldNamesStruct, HasRGB, HasAlpha)
% check types
if ~isa(XYZ, 'single')
    coder.internal.error('ros:slros2:pointcloud:InvalidXYZType', 'single');
elseif HasRGB && ~isa(RGB, 'double')
    coder.internal.error('ros:slros2:pointcloud:InvalidRGBType', 'double');
elseif HasAlpha && ~isa(Alpha, 'double')
    coder.internal.error('ros:slros2:pointcloud:InvalidAlphaType', 'double');
end
% check sizes   
unstructured = ismatrix(XYZ); 
if unstructured  
    if ~(size(XYZ, 2) == 3 && ismatrix(XYZ))
        coder.internal.error('ros:slros2:pointcloud:IncorrectSizeXYZ');
    elseif HasRGB && ~(size(RGB, 2) == 3 && ismatrix(RGB))
        coder.internal.error('ros:slros2:pointcloud:IncorrectSizeRGB');
    elseif HasAlpha && ~(size(Alpha, 2) == 1 && ismatrix(Alpha))
        coder.internal.error('ros:slros2:pointcloud:IncorrectSizeAlpha');
    elseif HasAlpha && ~(size(Alpha, 1) == size(RGB, 1))
        coder.internal.error('ros:slros2:pointcloud:IncompatibleSizesRGBAlpha');
    end
else % structured 
    if ~(size(XYZ, 3) == 3 && ~ismatrix(XYZ))
        coder.internal.error('ros:slros2:pointcloud:IncorrectSizeXYZ');
    elseif HasRGB && ~(size(RGB, 3) == 3 && ~ismatrix(RGB))
        coder.internal.error('ros:slros2:pointcloud:IncorrectSizeRGB');
    elseif HasAlpha && ~ismatrix(Alpha)
        coder.internal.error('ros:slros2:pointcloud:IncorrectSizeAlpha');
    elseif HasAlpha && ~(size(Alpha, 1) == size(RGB, 1) && size(Alpha, 2) == size(RGB, 2))
        coder.internal.error('ros:slros2:pointcloud:IncompatibleSizesRGBAlpha');
    end
end
if HasRGB && ~all(size(XYZ) == size(RGB))
    coder.internal.error('ros:slros2:pointcloud:IncompatibleSizesRGBXYZ');
end

if HasAlpha && unstructured
    RGBInput = cat(2, RGB, Alpha);
elseif HasAlpha
    RGBInput = cat(3, RGB, Alpha);
else
    RGBInput = RGB;
end
MaxDataLength = length(LidarMsgIn.data);
NumFields = length(LidarMsgIn.fields);
NameLength = length(LidarMsgIn.fields(1).name);
[Height, Width, FPFieldLengths, PointStep, ...
    RowStep, DataLength, Data, FPNames, ...
    FPNameLengths, FPOffsets, FPDatatypes, FPCounts] ...
    = ros.internal.block.WritePointCloudFncBlock(MaxDataLength, NumFields, NameLength, XYZ, RGBInput, FieldNamesStruct);
